simulink model "open_mha_drc_filter"  (R2020b)
settings: Solver=FixedStepDiscrete  StartTime=0.0  StopTime=stopTime  FixedStep=1.0416666666666666e-05  RelTol=1e-3
InitFcn:
  | initCallback
StopFcn:
  | stopCallback
settings Model: Creator=Ross  LastModifiedBy=conno
settings DataIOCC: SaveOutput=off  SaveTime=off  ReturnWorkspaceOutputs=off
settings OptimizationCC: BlockReduction=off  ConditionallyExecuteInputs=off  DefaultParameterBehavior=Inlined
settings DebuggingCC: ReadBeforeWriteMsg=DisableAll  WriteAfterWriteMsg=DisableAll  WriteAfterReadMsg=DisableAll  AlgebraicLoopMsg=error  MultiTaskDSMMsg=none  SingleTaskRateTransMsg=error  PregeneratedLibrarySubsystemCodeDiagnostic=none  ArithmeticOperatorsInVariantConditions=warning
settings HardwareCC: ProdBitPerPointer=32  ProdBitPerSizeT=32  ProdBitPerPtrDiffT=32  ProdLargestAtomicFloat=None  ProdIntDivRoundTo=Undefined  ProdEndianess=Unspecified  ProdWordSize=32  ProdHWDeviceType=ASIC/FPGA->ASIC/FPGA  TargetBitPerPointer=64  TargetBitPerSizeT=64  TargetBitPerPtrDiffT=64  TargetLongLongMode=on  TargetIntDivRoundTo=Zero  TargetEndianess=LittleEndian  TargetWordSize=64  TargetHWDeviceType=Custom Processor->MATLAB Host Computer  ProdEqTarget=off
settings ModelReferenceCC: UpdateModelReferenceTargets=IfOutOfDate
settings SFSimCC: SFSimEcho=off  SimUseLocalCustomCode=off  CustomCodeUndefinedFunction=UseInterfaceOnly
settings RTWCC: RTWUseLocalCustomCode=off

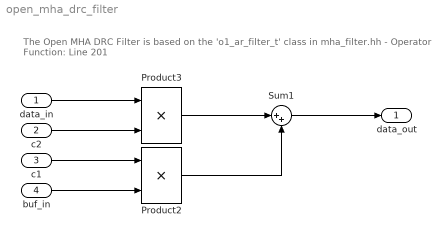
== system open_mha_drc_filter ==
  note: The Open MHA DRC Filter is based on the 'o1_ar_filter_t' class in mha_filter.hh
      | - Operator Function: Line 201
  data_in : Inport  OutDataTypeStr=fixdt(1,40,32)  PortDimensions=1  SampleTime=[1.0416666666666666e-05,0]
  c2 : Inport  Port=2  OutDataTypeStr=fixdt(0,16,16)  PortDimensions=1  SampleTime=[1.0416666666666666e-05,0]
  c1 : Inport  Port=3  OutDataTypeStr=fixdt(0,16,16)  PortDimensions=1  SampleTime=[1.0416666666666666e-05,0]
  buf_in : Inport  Port=4  OutDataTypeStr=fixdt(0,40,32)  PortDimensions=1  SampleTime=[1.0416666666666666e-05,0]
  Product2 : Product
  Product3 : Product
  Sum1 : Sum  Inputs=|++
  data_out : Outport  OutDataTypeStr=fixdt(1,58,48)  PortDimensions=1  SampleTime=[1.0416666666666666e-05,0]
  wires:
  Product3/1 -> Sum1/1
  Product2/1 -> Sum1/2
  Sum1/1 -> data_out/1
  c2/1 -> Product3/2
  buf_in/1 -> Product2/2
  c1/1 -> Product2/1
  data_in/1 -> Product3/1
